simulink model "position_control"  (R2021a)
settings: Solver=ode23t  StartTime=0.0  StopTime=200  RelTol=1e-5
values from neighbouring files (symbols this model uses):
  g = 9.81    [quad_params.m]
  I = [     0.005831943165131                   0                   0 ... (first row only)    [quad_params.m]
  Kd_rates = [0.05,0.05,0.1]'    [quad_params.m]
  Kd_vel = [0.8,0.8,0.3]'    [quad_params.m]
  Ki_vel = [0.1,0.1,0.1]'    [quad_params.m]
  km = 1.2e-7    (= 1.2e-07)    [quad_params.m]
  Kp_att = [6,6,6]'    [quad_params.m]
  Kp_pos = [7,7,3]'    [quad_params.m]
  Kp_rates = [10,10,10]'    [quad_params.m]
  Kp_vel = [3,3,5]'    [quad_params.m]
  kt = 0.9e-5    (= 9e-06)    [quad_params.m]
  L = 0.2    [quad_params.m]
  m = 0.9272    [quad_params.m]
  q_init = [1;0;0;0]    [quad_params.m]
  rate_p_max = 3.5    [quad_params.m]
  thrust_max = thrust_max_per_motor*4    (= 32)    [quad_params.m]
  thrust_max_per_motor = 8    [quad_params.m]
  tilt_max = pi/6    (= 0.523598775598)    [quad_params.m]
  TQ_max_per_motor = km*(w_max.^2)    [quad_params.m]
  Vb_init = [0;0;0]    [quad_params.m]
  vel_xy_max = 15    [quad_params.m]
  vel_z_max = 10    [quad_params.m]
  wb_init = [0;0;0]    [quad_params.m]
  Xe_init = [0;0;0]    [quad_params.m]
undefined symbols (not defined in the file or in its folder): pm_0, sigbuilder_block, Vm_0, X, xme_0, Y, Z
libraries: simulink_extras x16, nesl_utility x5, aerolibutil x4, sm_lib x4, simulink x3, pid_lib x3, sharedtransform x3, sharedutil x1, vrlib x1, aerolibanim x1
(part 1 of 3)
settings Model: Creator=Petronas-Tareq  LastModifiedBy=Petronas-Tareq
settings SolverCC: AutoInsertRateTranBlk=on  InsertRTBMode=Always

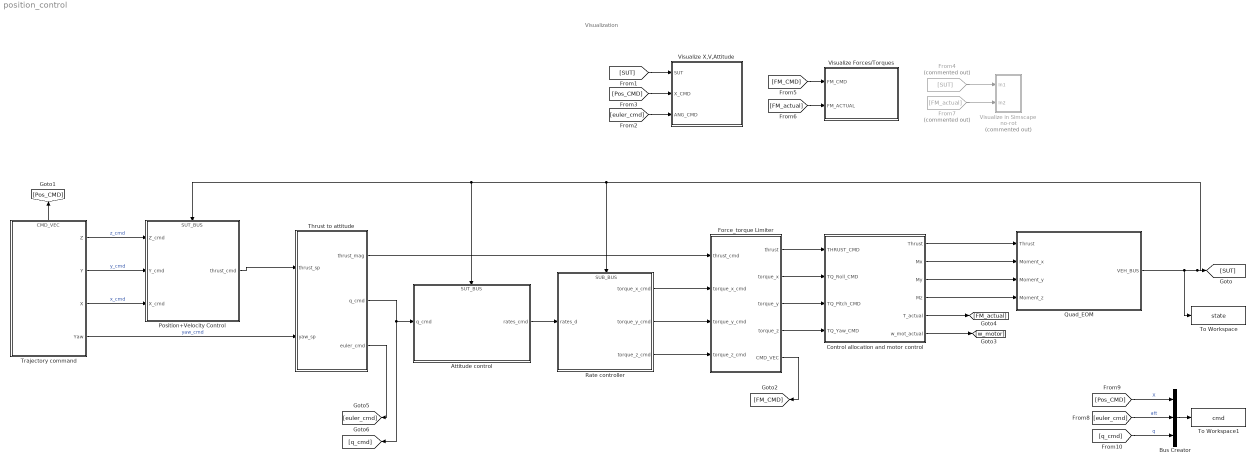
== system position_control ==
  note: Visualization
  Attitude control : Subsystem
      settings: PortSchema="{\"entries\":[{\"content\":{\"sides\":[{\"content\":{\"connectorIds\":[\"In1\"]},\"type\":\"ConnectorPlacement.EquallySpacedRectSide\",\"uuid\":\"19a574f6-5314-4727-8968-5b1c9712010e\"},{\"content\":{\"connectorIds\":[\"Out1\"],\"side\":\"RIGHT\"},\"type\":\"ConnectorPlacement.EquallySpacedRectSide\",\"uuid\":\"5cd6813f-6e17-48c1-918b-7c366c6d9cfa\"},{\"content\":{\"connectorIds\":[\"In2\"],\"side\":\"TOP\"},\"type\":\"ConnectorPlacement.EquallySpacedRectSide\",\"uuid\":\"b2bca67c-c4f4-4722-89a0-a16251073bfd\"}]},\"type\":\"ConnectorPlacement.EquallySpacedConnector\",\"uuid\":\"dcbf54f5-c136-40d5-a3db-9d2776e5196c\"}],\"packageUris\":[\"http://schema.mathworks.com/mf0/Connector/R2020b\"],\"version\":\"1.0\"}"
      mask Display: image('$imagefile'); % Use "Edit Image" on toolstrip to change.
  Bus Creator : BusCreator  Inputs=3
  Control allocation and motor control : Subsystem  Variant=on  VariantControlMode=label  LabelModeActiveChoice=Choice1
      mask Display: image('$imagefile'); % Use "Edit Image" on toolstrip to change.
  Force_torque Limiter : Subsystem
  From4 : From  Commented=on  GotoTag=SUT
  From7 : From  Commented=on  GotoTag=FM_actual
  Position+Velocity Control : Subsystem
      settings: PortSchema="{\"entries\":[{\"content\":{\"sides\":[{\"content\":{\"connectorIds\":[\"In1\",\"In2\",\"In3\"]},\"type\":\"ConnectorPlacement.EquallySpacedRectSide\",\"uuid\":\"cfe37ea9-b8e2-443a-9d65-596f0fda79c9\"},{\"content\":{\"connectorIds\":[\"Out1\"],\"side\":\"RIGHT\"},\"type\":\"ConnectorPlacement.EquallySpacedRectSide\",\"uuid\":\"f39f64e1-4b16-444a-b7d2-95ecb1b2a6fa\"},{\"content\":{\"connectorIds\":[\"In4\"],\"side\":\"TOP\"},\"type\":\"ConnectorPlacement.EquallySpacedRectSide\",\"uuid\":\"52402c3a-f2ac-44cf-8c94-dbfc3f851d2b\"}]},\"type\":\"ConnectorPlacement.EquallySpacedConnector\",\"uuid\":\"0122f56a-2702-493b-af7d-a25e6b9e04ed\"}],\"packageUris\":[\"http://schema.mathworks.com/mf0/Connector/R2020b\"],\"version\":\"1.0\"}"
  Quad_EOM : Subsystem
      mask Display: image('$imagefile'); % Use "Edit Image" on toolstrip to change.
  Rate controller : Subsystem
      settings: PortSchema="{\"entries\":[{\"content\":{\"sides\":[{\"content\":{\"connectorIds\":[\"In1\"]},\"type\":\"ConnectorPlacement.EquallySpacedRectSide\",\"uuid\":\"0af60e35-7b10-4750-a6af-1a3d920b4771\"},{\"content\":{\"connectorIds\":[\"Out1\",\"Out2\",\"Out3\"],\"side\":\"RIGHT\"},\"type\":\"ConnectorPlacement.EquallySpacedRectSide\",\"uuid\":\"931b0f34-b3f1-4a41-949f-3d763eca3151\"},{\"content\":{\"connectorIds\":[\"In2\"],\"side\":\"TOP\"},\"type\":\"ConnectorPlacement.EquallySpacedRectSide\",\"uuid\":\"84fe42fa-07d1-4fd9-ad2f-8c6651eaa98c\"}]},\"type\":\"ConnectorPlacement.EquallySpacedConnector\",\"uuid\":\"f603d2ac-5c20-4a82-ba8b-1c7971d6778a\"}],\"packageUris\":[\"http://schema.mathworks.com/mf0/Connector/R2020b\"],\"version\":\"1.0\"}"
  Thrust to attitude : Subsystem
  To Workspace : ToWorkspace  VariableName=state  SaveFormat=Timeseries  SampleTime=-1
  To Workspace1 : ToWorkspace  VariableName=cmd  SaveFormat=Timeseries  SampleTime=-1
  Trajectory command : Subsystem  Variant=on  VariantControlMode=label  LabelModeActiveChoice=6
      settings: PortSchema="{\"entries\":[{\"content\":{\"sides\":[{\"content\":{\"connectorIds\":[]},\"type\":\"ConnectorPlacement.EquallySpacedRectSide\",\"uuid\":\"8b658e99-682c-4d99-9859-63a6cdcf875c\"},{\"content\":{\"connectorIds\":[\"Out1\",\"Out2\",\"Out3\",\"Out4\"],\"side\":\"RIGHT\"},\"type\":\"ConnectorPlacement.EquallySpacedRectSide\",\"uuid\":\"566e7e32-52b1-45cc-9bb3-5343461c1cc0\"},{\"content\":{\"connectorIds\":[\"Out5\"],\"side\":\"TOP\"},\"type\":\"ConnectorPlacement.EquallySpacedRectSide\",\"uuid\":\"4cb1ab19-6483-4408-b5f4-106b35038f17\"}]},\"type\":\"ConnectorPlacement.EquallySpacedConnector\",\"uuid\":\"dc7c82fc-432d-4c18-9829-e6c2b483f5a7\"}],\"packageUris\":[\"http://schema.mathworks.com/mf0/Connector/R2020b\"],\"version\":\"1.0\"}"
  Visualize Forces/Torques : Subsystem
  Visualize X,V,Attitude : Subsystem
  Visualize in Simscape no-rot : Subsystem  Commented=on
  wires:
  [FM_CMD] -> Visualize Forces/Torques/1(FM_CMD)
  Force_torque Limiter/5(CMD_VEC) -> [FM_CMD]
  [FM_actual] -> Visualize Forces/Torques/2(FM_ACTUAL)
  Trajectory command/2(Y) -> Position+Velocity Control/2(Y_cmd)  "y_cmd"
  [SUT] -> Visualize X,V,Attitude/1(SUT)
  [Pos_CMD] -> Visualize X,V,Attitude/2(X_CMD)
  Trajectory command/3(X) -> Position+Velocity Control/3(X_cmd)  "x_cmd"
  Control allocation and motor control/1(Thrust) -> Quad_EOM/1(Thrust)
  Control allocation and motor control/2(Mx) -> Quad_EOM/2(Moment_x)
  Control allocation and motor control/3(My) -> Quad_EOM/3(Moment_y)
  Control allocation and motor control/4(Mz) -> Quad_EOM/4(Moment_z)
  Control allocation and motor control/5(T_actual) -> [FM_actual]
  Control allocation and motor control/6(w_mot_actual) -> [w_motor]
  Trajectory command/1(Z) -> Position+Velocity Control/1(Z_cmd)  "z_cmd"
  [euler_cmd] -> Visualize X,V,Attitude/3(ANG_CMD)
  From4/1 -> Visualize in Simscape no-rot/1(In1)
  From7/1 -> Visualize in Simscape no-rot/2(In2)
  Force_torque Limiter/4(torque_z) -> Control allocation and motor control/4(TQ_Yaw_CMD)
  Force_torque Limiter/3(torque_y) -> Control allocation and motor control/3(TQ_Pitch_CMD)
  Force_torque Limiter/2(torque_x) -> Control allocation and motor control/2(TQ_Roll_CMD)
  Force_torque Limiter/1(thrust) -> Control allocation and motor control/1(THRUST_CMD)
  Thrust to attitude/1(thrust_mag) -> Force_torque Limiter/1(thrust_cmd)
  Rate controller/2(torque_y_cmd) -> Force_torque Limiter/3(torque_y_cmd)
  Rate controller/3(torque_z_cmd) -> Force_torque Limiter/4(torque_z_cmd)
  Rate controller/1(torque_x_cmd) -> Force_torque Limiter/2(torque_x_cmd)
  Attitude control/1(rates_cmd) -> Rate controller/1(rates_d)
  Trajectory command/5(CMD_VEC) -> [Pos_CMD]
  Bus Creator/1 -> To Workspace1/1
  [Pos_CMD] -> Bus Creator/1  "X"
  [euler_cmd] -> Bus Creator/2  "att"
  [q_cmd] -> Bus Creator/3  "q"
  Thrust to attitude/2(q_cmd) -> Attitude control/1(q_cmd), [q_cmd]
  Thrust to attitude/3(euler_cmd) -> [euler_cmd]
  Trajectory command/4(Yaw) -> Thrust to attitude/2(yaw_sp)  "yaw_cmd"
  Position+Velocity Control/1(thrust_cmd) -> Thrust to attitude/1(thrust_sp)
  Quad_EOM/1(VEH_BUS) -> To Workspace/1, Rate controller/2(SUB_BUS), Position+Velocity Control/4(SUT_BUS), Attitude control/2(SUT_BUS), [SUT]

== system position_control/Attitude control ==
  note: Attitude control (full attitude control, i.e. yaw+thrust)
  note: Attitude Error Calculation
  q_cmd : Inport
  SUT_BUS : Inport  Port=2
  Bus Selector3 : BusSelector  OutputSignals=q
  K_attitude : Gain  Gain=Kp_att
  MATLAB Function1 : MATLAB Function  TreatAsAtomicUnit=on
  Product : Product
  Quaternion Inverse : aerolibutil/Quaternion Inverse
  Quaternion multiply : aerolibutil/Quaternion Multiplication
  Selector1 : Selector  InputPortWidth=4  IndexOptions=Index vector (dialog)  Indices=1  OutputSizes=1
  Selector2 : Selector  InputPortWidth=4  IndexOptions=Index vector (dialog)  Indices=2:4  OutputSizes=1
  k : Gain  Gain=2
  rates_cmd : Outport  VectorParamsAs1DForOutWhenUnconnected=off
  wires:
  SUT_BUS/1 -> [SUT]
  q_cmd/1 -> Quaternion multiply/2  "q_d"
  [SUT] -> Bus Selector3/1
  Bus Selector3/1 -> Quaternion Inverse/1  "<q>"
  Product/1 -> k/1  "error"
  Selector1/1 -> MATLAB Function1/1(q0)  "q0"
  MATLAB Function1/1(y) -> Product/1
  Selector2/1 -> Product/2  "q_vec"
  Quaternion multiply/1 -> Selector2/1, Selector1/1  "qe"
  k/1 -> K_attitude/1
  Quaternion Inverse/1 -> Quaternion multiply/1
  K_attitude/1 -> rates_cmd/1  "rates_cmd"

== system position_control/Control allocation and motor control ==
  note: 1) Add Subsystem or Model blocks as valid variant choices.
      | 2) You cannot connect blocks at this level. At simulation, connectivity is automatically
      | determined, based on the active variant and port name matching.
  THRUST_CMD : Inport
  TQ_Roll_CMD : Inport  Port=2
  TQ_Pitch_CMD : Inport  Port=3
  TQ_Yaw_CMD : Inport  Port=4
  Ideal Actuators with allocation : Subsystem  VariantControl=Choice2
  Ideal Actuattion (direct transfer) : Subsystem  VariantControl=Choice1
  Thrust : Outport
  Mx : Outport  Port=2
  My : Outport  Port=3
  Mz : Outport  Port=4
  T_actual : Outport  Port=5
  w_mot_actual : Outport  Port=6

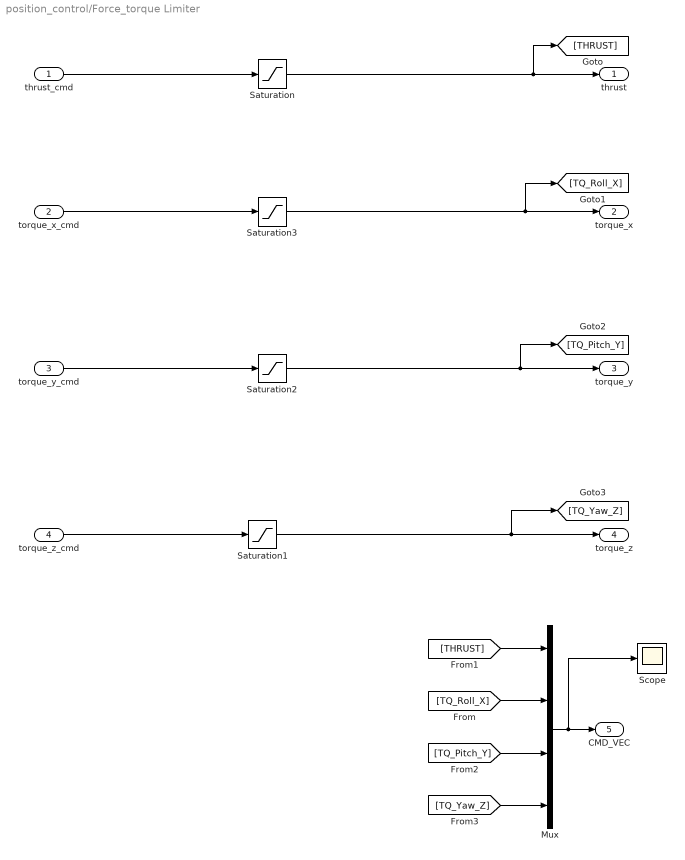
== system position_control/Force_torque Limiter ==
  thrust_cmd : Inport
  torque_x_cmd : Inport  Port=2
  torque_y_cmd : Inport  Port=3
  torque_z_cmd : Inport  Port=4
  Mux : Mux
  Saturation : Saturate  UpperLimit=thrust_max  LowerLimit=-thrust_max
      settings: AttributesFormatString=|
      | MAX =    %<UpperLimit>
      | MIN = %<LowerLimit>
  Saturation1 : Saturate  UpperLimit=2*TQ_max_per_motor  LowerLimit=-2*TQ_max_per_motor
      settings: AttributesFormatString=|
      | MAX =    %<UpperLimit>
      | MIN = %<LowerLimit>
  Saturation2 : Saturate  UpperLimit=thrust_max_per_motor*L  LowerLimit=-thrust_max_per_motor *L
      settings: AttributesFormatString=|
      | MAX =    %<UpperLimit>
      | MIN = %<LowerLimit>
  Saturation3 : Saturate  UpperLimit=thrust_max_per_motor*L  LowerLimit=-thrust_max_per_motor *L
      settings: AttributesFormatString=|
      | MAX =    %<UpperLimit>
      | MIN = %<LowerLimit>
  Scope : Scope
  thrust : Outport  VectorParamsAs1DForOutWhenUnconnected=off
  torque_x : Outport  Port=2  VectorParamsAs1DForOutWhenUnconnected=off
  torque_y : Outport  Port=3  VectorParamsAs1DForOutWhenUnconnected=off
  torque_z : Outport  Port=4  VectorParamsAs1DForOutWhenUnconnected=off
  CMD_VEC : Outport  Port=5  VectorParamsAs1DForOutWhenUnconnected=off
  wires:
  torque_z_cmd/1 -> Saturation1/1
  thrust_cmd/1 -> Saturation/1
  torque_y_cmd/1 -> Saturation2/1
  torque_x_cmd/1 -> Saturation3/1
  Saturation/1 -> [THRUST], thrust/1
  Saturation3/1 -> [TQ_Roll_X], torque_x/1
  Saturation2/1 -> [TQ_Pitch_Y], torque_y/1
  Saturation1/1 -> [TQ_Yaw_Z], torque_z/1
  Mux/1 -> Scope/1, CMD_VEC/1
  [THRUST] -> Mux/1
  [TQ_Roll_X] -> Mux/2
  [TQ_Pitch_Y] -> Mux/3
  [TQ_Yaw_Z] -> Mux/4

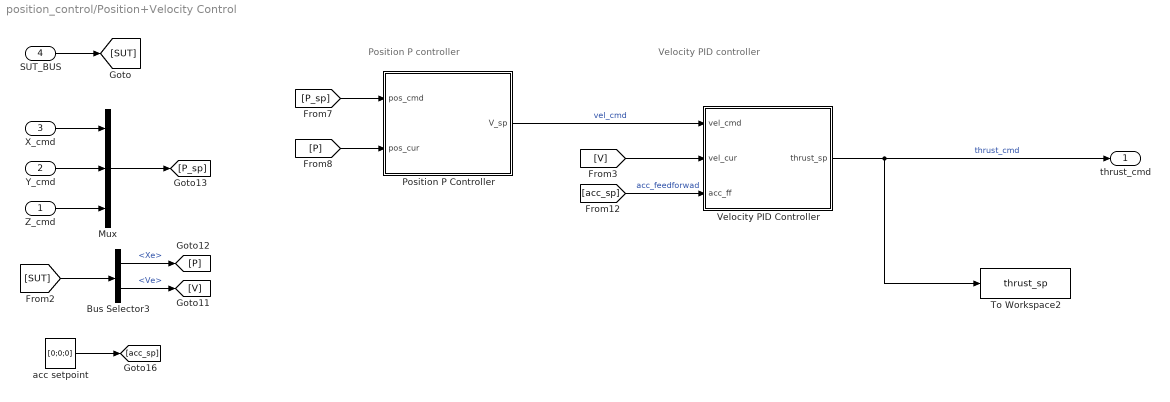
== system position_control/Position+Velocity Control ==
  note: Velocity PID controller
  note: Position P controller
  Z_cmd : Inport
  Y_cmd : Inport  Port=2
  X_cmd : Inport  Port=3
  SUT_BUS : Inport  Port=4
  Bus Selector3 : BusSelector  OutputSignals=Xe,Ve
  Mux : Mux  Inputs=3
  Position P Controller : Subsystem
  To Workspace2 : ToWorkspace  VariableName=thrust_sp  SaveFormat=Timeseries  SampleTime=-1
  Velocity PID Controller : Subsystem
  acc setpoint : Constant  Value=[0;0;0]
  thrust_cmd : Outport
  wires:
  SUT_BUS/1 -> [SUT]
  [SUT] -> Bus Selector3/1
  Bus Selector3/1 -> [P]  "<Xe>"
  Mux/1 -> [P_sp]
  acc setpoint/1 -> [acc_sp]
  [acc_sp] -> Velocity PID Controller/3(acc_ff)  "acc_feedforwad"
  Position P Controller/1(V_sp) -> Velocity PID Controller/1(vel_cmd)  "vel_cmd"
  [P_sp] -> Position P Controller/1(pos_cmd)
  [P] -> Position P Controller/2(pos_cur)
  [V] -> Velocity PID Controller/2(vel_cur)
  Velocity PID Controller/1(thrust_sp) -> To Workspace2/1, thrust_cmd/1  "thrust_cmd"
  Bus Selector3/2 -> [V]  "<Ve>"
  Z_cmd/1 -> Mux/3
  X_cmd/1 -> Mux/1
  Y_cmd/1 -> Mux/2

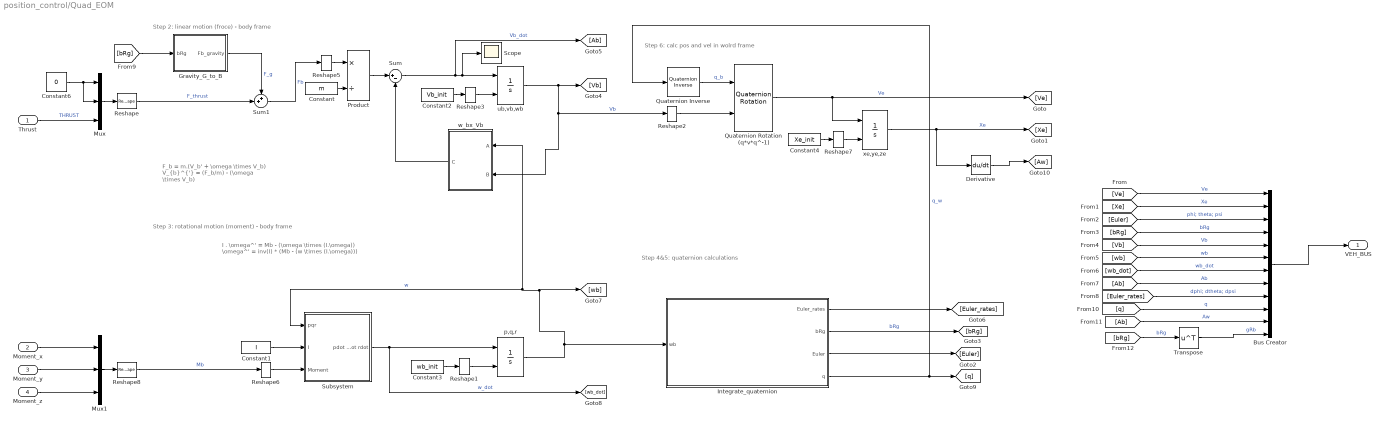
== system position_control/Quad_EOM ==
  note: Step 3: rotational motion (moment) - body frame
  note: F_b = m.(V_b' + \omega \times V_b)
      |
      | V_{b}^{'} = (F_b/m) - (\omega \times V_b)
  note: Step 2: linear motion (froce) - body frame
  note: Step 6: calc pos and vel in wolrd frame
  note: I . \omega^' = Mb - (\omega \times (I.\omega))
      |
      | \omega^' = inv(I) * (Mb - (w \times (I.\omega)))
  note: Step 4&5: quaternion calculations
  Thrust : Inport
  Moment_x : Inport  Port=2
  Moment_y : Inport  Port=3
  Moment_z : Inport  Port=4
  Bus Creator : BusCreator  Inputs=12
  Constant : Constant  Value=m  OutDataTypeStr=Inherit: Inherit via back propagation
  Constant1 : Constant  Value=I  OutDataTypeStr=Inherit: Inherit via back propagation
  Constant2 : Constant  Value=Vb_init  OutDataTypeStr=Inherit: Inherit via back propagation
  Constant3 : Constant  Value=wb_init  OutDataTypeStr=Inherit: Inherit via back propagation
  Constant4 : Constant  Value=Xe_init  OutDataTypeStr=Inherit: Inherit via back propagation
  Constant6 : Constant  Value=0
  Derivative : Derivative
  Gravity_G_to_B : Subsystem
  Integrate_quaternion : Subsystem
  Mux : Mux  Inputs=3
  Mux1 : Mux  Inputs=3
  Product : Product  Inputs=*/  SaturateOnIntegerOverflow=on  OutDataTypeStr=Inherit: Same as first input
  Quaternion Inverse : aerolibutil/Quaternion Inverse
  Quaternion Rotation (q*v*q^-1) : aerolibutil/Quaternion Rotation
  Reshape{,1..3,5..8} (8 alike) : Reshape  OutputDimensionality=Column vector (2-D)
  Scope : Scope
  Subsystem : Subsystem
  Sum : Sum  Inputs=|+-  SaturateOnIntegerOverflow=on
  Sum1 : Sum  Inputs=++|
  Transpose : Math  Operator=transpose  SaturateOnIntegerOverflow=on
  "p,q,r " : Integrator  InitialConditionSource=external  InitialCondition=pm_0
  ub,vb,wb : Integrator  InitialConditionSource=external  InitialCondition=Vm_0
  w_bx_Vb : Subsystem
      mask Display:
      | text(.5,.5,'Cross\nProduct\n\nC = AxB', ...
      | 	'HorizontalAlignment','Center',...
      | 	'VerticalAlignment','middle')
  xe,ye,ze : Integrator  InitialConditionSource=external  InitialCondition=xme_0
  VEH_BUS : Outport  VectorParamsAs1DForOutWhenUnconnected=off
  wires:
  [Euler] -> Bus Creator/3  "phi; theta; psi"
  [Xe] -> Bus Creator/2  "Xe"
  [Ve] -> Bus Creator/1  "Ve"
  [bRg] -> Bus Creator/4  "bRg"
  [Ab] -> Bus Creator/8  "Ab"
  [wb_dot] -> Bus Creator/7  "wb_dot"
  Bus Creator/1 -> VEH_BUS/1
  [Vb] -> Bus Creator/5  "Vb"
  [wb] -> Bus Creator/6  "wb"
  [Euler_rates] -> Bus Creator/9  "dphi; dtheta; dpsi"
  Reshape8/1 -> Reshape6/1  "Mb"
  Reshape6/1 -> Subsystem/3(Moment)
  Reshape1/1 -> "p,q,r "/2
  Constant2/1 -> Reshape3/1
  Subsystem/1(pdot qdot rdot) -> [wb_dot], "p,q,r "/1  "w_dot"
  Constant/1 -> Product/2
  Constant1/1 -> Subsystem/2(I)
  w_bx_Vb/1(C) -> Sum/2
  Integrate_quaternion/2(bRg) -> [bRg]  "bRg"
  Sum/1 -> [Ab], Scope/1, ub,vb,wb/1  "Vb_dot"
  Constant4/1 -> Reshape7/1
  Reshape3/1 -> ub,vb,wb/2
  Reshape7/1 -> xe,ye,ze/2
  Quaternion Rotation (q*v*q^-1)/1 -> xe,ye,ze/1, [Ve]  "Ve"
  Reshape5/1 -> Product/1
  xe,ye,ze/1 -> Derivative/1, [Xe]  "Xe"
  Sum1/1 -> Reshape5/1  "Fb"
  Constant3/1 -> Reshape1/1
  Product/1 -> Sum/1
  Constant6/1 -> Mux/2, Mux/1
  Gravity_G_to_B/1(Fb_gravity) -> Sum1/1  "F_g"
  Mux/1 -> Reshape/1
  Reshape/1 -> Sum1/2  "F_thrust"
  Thrust/1 -> Mux/3  "THRUST"
  [bRg] -> Gravity_G_to_B/1(bRg)
  Moment_y/1 -> Mux1/2
  Moment_z/1 -> Mux1/3
  Mux1/1 -> Reshape8/1
  Moment_x/1 -> Mux1/1
  "p,q,r "/1 -> [wb], Subsystem/1(pqr), w_bx_Vb/1(A), Integrate_quaternion/1(wb)  "w"
  ub,vb,wb/1 -> [Vb], w_bx_Vb/2(B), Reshape2/1  "Vb"
  Integrate_quaternion/1(Euler_rates) -> [Euler_rates]
  Integrate_quaternion/3(Euler) -> [Euler]
  [q] -> Bus Creator/10  "q"
  Integrate_quaternion/4(q) -> Quaternion Inverse/1, [q]  "q_w"
  Reshape2/1 -> Quaternion Rotation (q*v*q^-1)/2
  Quaternion Inverse/1 -> Quaternion Rotation (q*v*q^-1)/1  "q_b"
  Derivative/1 -> [Aw]
  [Ab] -> Bus Creator/11  "Aw"
  [bRg] -> Transpose/1  "bRg"
  Transpose/1 -> Bus Creator/12  "gRb"

== system position_control/Rate controller ==
  note: Rate controller
  rates_d : Inport
  SUB_BUS : Inport  Port=2
  Bus Selector1 : BusSelector  OutputSignals=wb,wb_dot
  Demux : Demux  Outputs=3
  Kd_rates : Gain  Gain=Kd_rates
  Kp_rates : Gain  Gain=Kp_rates
  Scope : Scope  NumInputPorts=2
  Sum : Sum  Inputs=|+-
  Sum1 : Sum  Inputs=|+-
  limit rate p : Saturate  UpperLimit=rate_p_max  LowerLimit=-rate_p_max
  limit rate q : Saturate  UpperLimit=rate_p_max  LowerLimit=-rate_p_max
  limit rate r : Saturate  UpperLimit=rate_p_max  LowerLimit=-rate_p_max
  torque_x_cmd : Outport
  torque_y_cmd : Outport  Port=2
  torque_z_cmd : Outport  Port=3
  wires:
  Bus Selector1/2 -> Kd_rates/1  "<wb_dot>"
  Bus Selector1/1 -> Sum1/2, Scope/2  "<wb>"
  Demux/1 -> limit rate p/1
  Demux/2 -> limit rate q/1
  Demux/3 -> limit rate r/1
  SUB_BUS/1 -> Bus Selector1/1  "measurements"
  rates_d/1 -> Sum1/1, Scope/1
  Kd_rates/1 -> Sum/2  "w_d"
  Kp_rates/1 -> Sum/1
  Sum/1 -> Demux/1  "torques"
  Sum1/1 -> Kp_rates/1
  limit rate p/1 -> torque_x_cmd/1
  limit rate q/1 -> torque_y_cmd/1
  limit rate r/1 -> torque_z_cmd/1

== system position_control/Thrust to attitude ==
  note: Thrust vector and Yaw to Attitude and total Thrust
  thrust_sp : Inport
  yaw_sp : Inport  Port=2
  Bus Creator : BusCreator  Inputs=3
  Demux4 : Demux  Outputs=3
  Direction Cosine Matrix to Quaternions : sharedtransform/Direction Cosine Matrix  to Quaternions  aMode=0  action=None  tolerance=eps(2)
      settings: SourceProductBaseCode=AE,PW,DR,MT,UV,VE
  MATLAB Function4 : MATLAB Function  TreatAsAtomicUnit=on
  Quaternions to Rotation Angles : sharedtransform/Quaternions to Rotation Angles  rotationOrder=ZYX  aMode=aMode
      settings: SourceProductBaseCode=AE,PW,DR,MT,UV,VE
  Scope1 : Scope
  Scope2 : Scope
  Subsystem : Subsystem  Commented=on
  To Workspace : ToWorkspace  VariableName=thrust_unit_dir  SaveFormat=Timeseries  SampleTime=-1
  To Workspace1 : ToWorkspace  VariableName=thrust_mag  SaveFormat=Timeseries  SampleTime=-1
  thrust_mag : Outport
  q_cmd : Outport  Port=2
  euler_cmd : Outport  Port=3
  wires:
  thrust_sp/1 -> Scope1/1, MATLAB Function4/1(thrust_sp)  "thrust_cmd"
  MATLAB Function4/1(R_sp) -> To Workspace/1, Direction Cosine Matrix to Quaternions/1
  MATLAB Function4/2(thrust_mag) -> thrust_mag/1, To Workspace1/1
  Direction Cosine Matrix to Quaternions/1 -> q_cmd/1, Quaternions to Rotation Angles/1
  yaw_sp/1 -> MATLAB Function4/2(yaw_sp)  "yaw_cmd"
  Demux4/1 -> Bus Creator/1  "yaw"
  Demux4/3 -> Bus Creator/3  "roll"
  Bus Creator/1 -> Scope2/1, euler_cmd/1
  Demux4/2 -> Bus Creator/2  "pitch"
  Quaternions to Rotation Angles/1 -> Demux4/1

== system position_control/Trajectory command ==
  Altitude : Subsystem  VariantControl=1
  Ground : Subsystem  VariantControl=0
  Position Trajectory : Subsystem  VariantControl=5
  Test to visualize thrust dir : Subsystem  VariantControl=6
  X Sine : Subsystem  VariantControl=4
  X ramp : Subsystem  VariantControl=9
  X square : Subsystem  VariantControl=7
  Y Sine : Subsystem  VariantControl=3
  Y ramp : Subsystem  VariantControl=8
  Yaw Sine : Subsystem  VariantControl=2
  Z : Outport
  Y : Outport  Port=2
  X : Outport  Port=3
  Yaw : Outport  Port=4
  CMD_VEC : Outport  Port=5

== system position_control/Visualize Forces//Torques ==
  FM_CMD : Inport
  FM_ACTUAL : Inport  Port=2
  FM CMD vs Actual : Scope  NumInputPorts=4
  FM_Mux : Subsystem
  wires:
  FM_CMD/1 -> [FM_CMD]
  [FM_CMD] -> FM_Mux/1(FM_CMD)
  [FM] -> FM_Mux/2(FM)
  FM_Mux/1(Y1) -> FM CMD vs Actual/1  "Thrust"
  FM_Mux/2(Y2) -> FM CMD vs Actual/2  "TQ_Roll_X"
  FM_Mux/3(w3) -> FM CMD vs Actual/3  "TQ_Pitch_Y"
  FM_Mux/4(Y4) -> FM CMD vs Actual/4  "TQ_Yaw_Z"
  FM_ACTUAL/1 -> [FM]

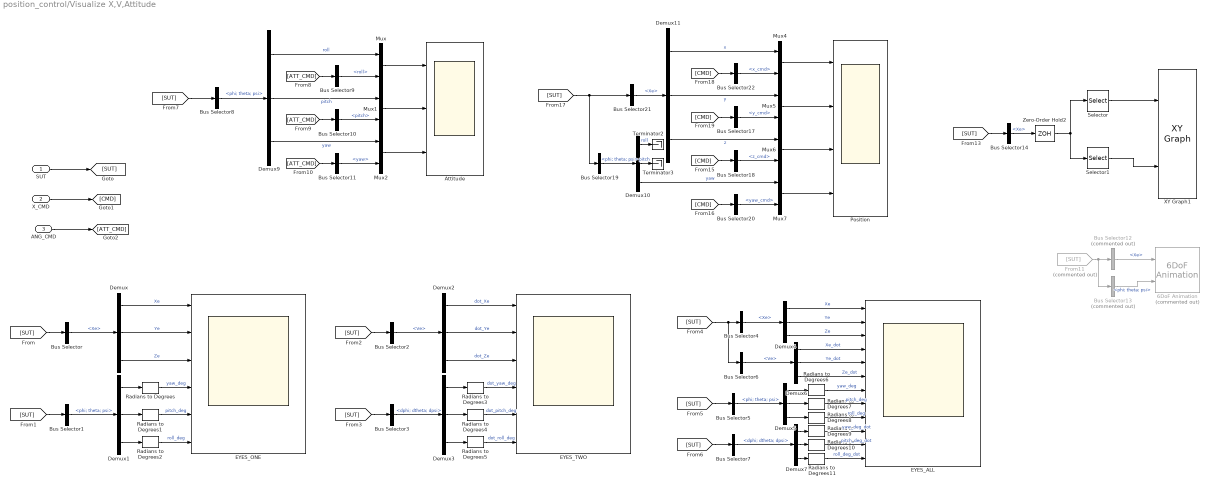
== system position_control/Visualize X,V,Attitude ==
  SUT : Inport
  X_CMD : Inport  Port=2
  ANG_CMD : Inport  Port=3
  6DoF Animation : aerolibanim/6DoF Animation  Commented=on  u1=[-20 20 -20 20 -20 20]  u2=0.05  u3=0.5  u4=[-5 -5 0 5]  u5=Fly alongside  u6=[0 0 0]  u7=10  u8=on
  "Attitude " : Scope  NumInputPorts=3
  Bus Selector{,4,14,21} (4 alike) : BusSelector  OutputSignals=Xe
  Bus Selector{1,5,8,19} (4 alike) : BusSelector  OutputSignals=phi; theta; psi
  Bus Selector10 : BusSelector  OutputSignals=pitch
  Bus Selector11 : BusSelector  OutputSignals=yaw
  Bus Selector12 : BusSelector  Commented=on  OutputSignals=Xe
  Bus Selector13 : BusSelector  Commented=on  OutputSignals=phi; theta; psi
  Bus Selector17 : BusSelector  OutputSignals=y_cmd
  Bus Selector18 : BusSelector  OutputSignals=z_cmd
  Bus Selector2 : BusSelector  OutputSignals=Ve
  Bus Selector20 : BusSelector  OutputSignals=yaw_cmd
  Bus Selector22 : BusSelector  OutputSignals=x_cmd
  Bus Selector3 : BusSelector  OutputSignals=dphi; dtheta; dpsi
  Bus Selector6 : BusSelector  OutputSignals=Ve
  Bus Selector7 : BusSelector  OutputSignals=dphi; dtheta; dpsi
  Bus Selector9 : BusSelector  OutputSignals=roll
  Demux{,1..7,9..11} (11 alike) : Demux  Outputs=3
  EYES_ALL : Scope  NumInputPorts=12
  EYES_ONE : Scope  NumInputPorts=6
  EYES_TWO : Scope  NumInputPorts=6
  From11 : From  Commented=on  GotoTag=SUT
  Mux{,1..2,4..7} (7 alike) : Mux  Inputs=2
  Position : Scope  NumInputPorts=4
  Radians to Degrees{,1..11} (12 alike) : simulink_extras/Transformations/Radians to Degrees
  Selector : Selector  InputPortWidth=3  IndexOptions=Index vector (dialog)  Indices=1  OutputSizes=1
  Selector1 : Selector  InputPortWidth=3  IndexOptions=Index vector (dialog)  Indices=2  OutputSizes=1
  Terminator2 : Terminator
  Terminator3 : Terminator
  XY Graph1 : simulink/Sinks/XY Graph  xmin=-1  xmax=30  ymin=-1  ymax=35  st=-1
  Zero-Order Hold2 : ZeroOrderHold  SampleTime=0.1
  wires:
  SUT/1 -> [SUT]
  [SUT] -> Bus Selector/1
  Demux/2 -> EYES_ONE/2  "Ye"
  Demux/3 -> EYES_ONE/3  "Ze"
  Demux/1 -> EYES_ONE/1  "Xe"
  Bus Selector/1 -> Demux/1  "<Xe>"
  Bus Selector1/1 -> Demux1/1  "<phi; theta; psi>"
  [SUT] -> Bus Selector1/1
  Demux1/1 -> Radians to Degrees/1
  Radians to Degrees/1 -> EYES_ONE/4  "yaw_deg"
  Radians to Degrees1/1 -> EYES_ONE/5  "pitch_deg"
  Radians to Degrees2/1 -> EYES_ONE/6  "roll_deg"
  Demux1/3 -> Radians to Degrees2/1
  Demux1/2 -> Radians to Degrees1/1
  [SUT] -> Bus Selector2/1
  Demux2/2 -> EYES_TWO/2  "dot_Ye"
  Demux2/3 -> EYES_TWO/3  "dot_Ze"
  Demux2/1 -> EYES_TWO/1  "dot_Xe"
  Bus Selector2/1 -> Demux2/1  "<Ve>"
  Bus Selector3/1 -> Demux3/1  "<dphi; dtheta; dpsi>"
  [SUT] -> Bus Selector3/1
  Demux3/1 -> Radians to Degrees3/1
  Radians to Degrees3/1 -> EYES_TWO/4  "dot_yaw_deg"
  Radians to Degrees4/1 -> EYES_TWO/5  "dot_pitch_deg"
  Radians to Degrees5/1 -> EYES_TWO/6  "dot_roll_deg"
  Demux3/3 -> Radians to Degrees5/1
  Demux3/2 -> Radians to Degrees4/1
  [SUT] -> Bus Selector6/1, Bus Selector4/1
  Demux4/2 -> EYES_ALL/2  "Ye"
  Demux4/3 -> EYES_ALL/3  "Ze"
  Demux4/1 -> EYES_ALL/1  "Xe"
  Bus Selector4/1 -> Demux4/1  "<Xe>"
  Bus Selector5/1 -> Demux5/1  "<phi; theta; psi>"
  [SUT] -> Bus Selector5/1
  Demux5/1 -> Radians to Degrees6/1
  Demux6/1 -> EYES_ALL/4  "Xe_dot"
  Demux6/2 -> EYES_ALL/5  "Ye_dot"
  Demux6/3 -> EYES_ALL/6  "Ze_dot"
  Demux5/3 -> Radians to Degrees8/1
  Demux5/2 -> Radians to Degrees7/1
  Bus Selector6/1 -> Demux6/1  "<Ve>"
  Radians to Degrees6/1 -> EYES_ALL/7  "yaw_deg"
  Radians to Degrees7/1 -> EYES_ALL/8  "pitch_deg"
  Radians to Degrees8/1 -> EYES_ALL/9  "roll_deg"
  Bus Selector7/1 -> Demux7/1  "<dphi; dtheta; dpsi>"
  [SUT] -> Bus Selector7/1
  Demux7/1 -> Radians to Degrees9/1
  Demux7/2 -> Radians to Degrees10/1
  Demux7/3 -> Radians to Degrees11/1
  Radians to Degrees9/1 -> EYES_ALL/10  "yaw_deg_dot"
  Radians to Degrees10/1 -> EYES_ALL/11  "pitch_deg_dot"
  Radians to Degrees11/1 -> EYES_ALL/12  "roll_deg_dot"
  X_CMD/1 -> [CMD]
  [SUT] -> Bus Selector8/1
  Demux9/2 -> Mux1/1  "pitch"
  Demux9/1 -> Mux/1  "roll"
  Bus Selector8/1 -> Demux9/1  "<phi; theta; psi>"
  Mux/1 -> "Attitude "/1
  Mux1/1 -> "Attitude "/2
  Mux2/1 -> "Attitude "/3
  Demux9/3 -> Mux2/1  "yaw"
  [ATT_CMD] -> Bus Selector9/1
  Bus Selector9/1 -> Mux/2  "<roll>"
  [ATT_CMD] -> Bus Selector10/1
  Bus Selector10/1 -> Mux1/2  "<pitch>"
  [ATT_CMD] -> Bus Selector11/1
  Bus Selector11/1 -> Mux2/2  "<yaw>"
  [SUT] -> Bus Selector14/1
  Bus Selector14/1 -> Zero-Order Hold2/1  "<Xe>"
  Zero-Order Hold2/1 -> Selector1/1, Selector/1
  Demux10/3 -> Mux7/1  "yaw"
  Mux7/1 -> Position/4
  Demux11/1 -> Mux4/1  "x"
  [CMD] -> Bus Selector20/1
  Bus Selector20/1 -> Mux7/2  "<yaw_cmd>"
  [CMD] -> Bus Selector17/1
  [SUT] -> Bus Selector21/1, Bus Selector19/1
  Demux10/2 -> Terminator3/1  "pitch"
  Mux6/1 -> Position/3
  Bus Selector19/1 -> Demux10/1  "<phi; theta; psi>"
  Demux10/1 -> Terminator2/1  "roll"
  Demux11/2 -> Mux5/1  "y"
  Bus Selector17/1 -> Mux5/2  "<y_cmd>"
  Mux4/1 -> Position/1
  Demux11/3 -> Mux6/1  "z"
  [CMD] -> Bus Selector22/1
  Mux5/1 -> Position/2
  Bus Selector22/1 -> Mux4/2  "<x_cmd>"
  Bus Selector18/1 -> Mux6/2  "<z_cmd>"
  [CMD] -> Bus Selector18/1
  Bus Selector21/1 -> Demux11/1  "<Xe>"
  ANG_CMD/1 -> [ATT_CMD]
  Selector/1 -> XY Graph1/1
  Selector1/1 -> XY Graph1/2
  From11/1 -> Bus Selector13/1, Bus Selector12/1
  Bus Selector12/1 -> 6DoF Animation/1  "<Xe>"
  Bus Selector13/1 -> 6DoF Animation/2  "<phi; theta; psi>"

== system position_control/Visualize in Simscape no-rot ==
  In1 : Inport
  In2 : Inport  Port=2
  6-DOF Joint1 : sm_lib/Joints/6-DOF Joint  JointMode=Normal  SenseConstraintForce=off  SenseConstraintForceX=off  SenseConstraintForceY=off  SenseConstraintForceZ=off  SenseConstraintTorque=off  SenseConstraintTorqueX=off  SenseConstraintTorqueY=off  SenseConstraintTorqueZ=off  SenseTotalForce=off  SenseTotalForceX=off  SenseTotalForceY=off  SenseTotalForceZ=off  SenseTotalTorque=off  SenseTotalTorqueX=off  SenseTotalTorqueY=off  SenseTotalTorqueZ=off  CompositeWrenchDir=FollowerOnBase  CompositeWrenchFrame=BaseFrame  PxEquilibriumPosition=0  PxEquilibriumPositionUnits=m  PxSpringStiffness=0  PxSpringStiffnessUnits=N/m  PxDampingCoefficient=0  PxDampingCoefficientUnits=N/(m/s)  PxTorqueActuationMode=ComputedTorque  PxMotionActuationMode=InputMotion  PxSensePosition=off  PxSenseVelocity=off  PxSenseAcceleration=off  PxSenseTorqueForce=off  PxSenseLowerLimitTorqueForce=off  PxSenseUpperLimitTorqueForce=off  PxLowerLimitSpecify=off  PxLowerLimitBound=-1  PxLowerLimitBoundUnits=m  PxLowerLimitStiffness=1e6  PxLowerLimitStiffnessUnits=N/m  PxLowerLimitDamping=1e3  PxLowerLimitDampingUnits=N/(m/s)  PxLowerLimitTransitionRegionWidth=1e-4  PxLowerLimitTransitionRegionWidthUnits=m  PxUpperLimitSpecify=off  PxUpperLimitBound=1  PxUpperLimitBoundUnits=m  PxUpperLimitStiffness=1e6  PxUpperLimitStiffnessUnits=N/m  PxUpperLimitDamping=1e3  PxUpperLimitDampingUnits=N/(m/s)  PxUpperLimitTransitionRegionWidth=1e-4  PxUpperLimitTransitionRegionWidthUnits=m  PxPositionTargetSpecify=on  PxPositionTargetPriority=High  PxPositionTargetValue=Xe_init(1)  PxPositionTargetValueUnits=m  PxVelocityTargetSpecify=off  PxVelocityTargetPriority=High  PxVelocityTargetValue=0  PxVelocityTargetValueUnits=m/s  PyEquilibriumPosition=0  PyEquilibriumPositionUnits=m  PySpringStiffness=0  PySpringStiffnessUnits=N/m  PyDampingCoefficient=0  PyDampingCoefficientUnits=N/(m/s)  PyTorqueActuationMode=ComputedTorque  PyMotionActuationMode=InputMotion  PySensePosition=off  PySenseVelocity=off  PySenseAcceleration=off  PySenseTorqueForce=off  PySenseLowerLimitTorqueForce=off  PySenseUpperLimitTorqueForce=off  PyLowerLimitSpecify=off  PyLowerLimitBound=-1  PyLowerLimitBoundUnits=m  PyLowerLimitStiffness=1e6  PyLowerLimitStiffnessUnits=N/m  PyLowerLimitDamping=1e3  PyLowerLimitDampingUnits=N/(m/s)  PyLowerLimitTransitionRegionWidth=1e-4  PyLowerLimitTransitionRegionWidthUnits=m  PyUpperLimitSpecify=off  PyUpperLimitBound=1  PyUpperLimitBoundUnits=m  PyUpperLimitStiffness=1e6  PyUpperLimitStiffnessUnits=N/m  PyUpperLimitDamping=1e3  PyUpperLimitDampingUnits=N/(m/s)  PyUpperLimitTransitionRegionWidth=1e-4  PyUpperLimitTransitionRegionWidthUnits=m  PyPositionTargetSpecify=on  PyPositionTargetPriority=High  PyPositionTargetValue=Xe_init(2)  PyPositionTargetValueUnits=m  PyVelocityTargetSpecify=off  PyVelocityTargetPriority=High  PyVelocityTargetValue=0  PyVelocityTargetValueUnits=m/s  PzEquilibriumPosition=0  PzEquilibriumPositionUnits=m  PzSpringStiffness=0  PzSpringStiffnessUnits=N/m  PzDampingCoefficient=0  PzDampingCoefficientUnits=N/(m/s)  PzTorqueActuationMode=ComputedTorque  PzMotionActuationMode=InputMotion  PzSensePosition=off  PzSenseVelocity=off  PzSenseAcceleration=off  PzSenseTorqueForce=off  PzSenseLowerLimitTorqueForce=off  PzSenseUpperLimitTorqueForce=off  PzLowerLimitSpecify=off  PzLowerLimitBound=-1  PzLowerLimitBoundUnits=m  PzLowerLimitStiffness=1e6  PzLowerLimitStiffnessUnits=N/m  PzLowerLimitDamping=1e3  PzLowerLimitDampingUnits=N/(m/s)  PzLowerLimitTransitionRegionWidth=1e-4  PzLowerLimitTransitionRegionWidthUnits=m  PzUpperLimitSpecify=off  PzUpperLimitBound=1  PzUpperLimitBoundUnits=m  PzUpperLimitStiffness=1e6  PzUpperLimitStiffnessUnits=N/m  PzUpperLimitDamping=1e3  PzUpperLimitDampingUnits=N/(m/s)  PzUpperLimitTransitionRegionWidth=1e-4  PzUpperLimitTransitionRegionWidthUnits=m  PzPositionTargetSpecify=on  PzPositionTargetPriority=High  PzPositionTargetValue=Xe_init(3)  PzPositionTargetValueUnits=m  PzVelocityTargetSpecify=off  PzVelocityTargetPriority=High  PzVelocityTargetValue=0  PzVelocityTargetValueUnits=m/s  SphDefPosRotationMethod=None  SphDefPosRotationAngleUnits=deg  SphDefPosRotationStandardAxis=+Z  SphDefPosRotationAngle=0.0  SphDefPosRotationArbitraryAxis=[0 0 1]  SphDefPosFollAlignAxisA=+X  SphDefPosBaseAlignAxisA=+Y  SphDefPosFollAlignAxisB=+Y  SphDefPosBaseAlignAxisB=+Z  SphDefPosRotationSequenceAxes=FollowerAxes  SphDefPosRotationSequence=XYX  SphDefPosRotationSequenceAngles=[0 0 0]  SphDefPosRotationSequenceAnglesUnits=deg  SphDefPosRotationMatrix=[1 0 0; 0 1 0; 0 0 1]  SphEqPosRotationMethod=None  SphEqPosRotationAngleUnits=deg  SphEqPosRotationStandardAxis=+Z  SphEqPosRotationAngle=0.0  SphEqPosRotationArbitraryAxis=[0 0 1]  SphEqPosFollAlignAxisA=+X  SphEqPosBaseAlignAxisA=+Y  SphEqPosFollAlignAxisB=+Y  SphEqPosBaseAlignAxisB=+Z  SphEqPosRotationSequenceAxes=FollowerAxes  SphEqPosRotationSequence=XYX  SphEqPosRotationSequenceAngles=[0 0 0]  SphEqPosRotationSequenceAnglesUnits=deg  SphEqPosRotationMatrix=[1 0 0; 0 1 0; 0 0 1]  SphSpringStiffness=0  SphSpringStiffnessUnits=N*m/deg  SphDampingCoefficient=0  SphDampingCoefficientUnits=N*m/(deg/s)  SphActuateTorqueX=off  SphActuateTorqueY=off  SphActuateTorqueZ=off  SphActuateTorque=on  SphTorqueActuationMode=InputTorque  SphMotionActuationMode=ComputedMotion  SphActuationFrame=BaseFrame  SphSensePosition=off  SphSenseVelocityX=off  SphSenseVelocityY=off  SphSenseVelocityZ=off  SphSenseVelocity=off  SphSenseAccelerationX=off  SphSenseAccelerationY=off  SphSenseAccelerationZ=off  SphSenseAcceleration=off  SphSenseTorqueX=off  SphSenseTorqueY=off  SphSenseTorqueZ=off  SphSenseTorqueForce=off  SphSenseLowerLimitTorqueMag=off  SphSenseUpperLimitTorqueMag=off  SphSensingFrame=BaseFrame  SphLowerLimitSpecify=off  SphLowerLimitBound=15  SphLowerLimitBoundUnits=deg  SphLowerLimitStiffness=1e4  SphLowerLimitStiffnessUnits=N*m/deg  SphLowerLimitDamping=10  SphLowerLimitDampingUnits=N*m/(deg/s)  SphLowerLimitTransitionRegionWidth=0.1  SphLowerLimitTransitionRegionWidthUnits=deg  SphUpperLimitSpecify=off  SphUpperLimitBound=45  SphUpperLimitBoundUnits=deg  SphUpperLimitStiffness=1e4  SphUpperLimitStiffnessUnits=N*m/deg  SphUpperLimitDamping=10  SphUpperLimitDampingUnits=N*m/(deg/s)  SphUpperLimitTransitionRegionWidth=0.1  SphUpperLimitTransitionRegionWidthUnits=deg  SphPositionTargetRotationMethod=RotationSequence  SphPositionTargetRotationAngleUnits=deg  SphPositionTargetRotationStandardAxis=+Z  SphPositionTargetRotationAngle=0.0  SphPositionTargetRotationArbitraryAxis=[0 0 1]  SphPositionTargetFollAlignAxisA=+X  SphPositionTargetBaseAlignAxisA=+Y  SphPositionTargetFollAlignAxisB=+Y  SphPositionTargetBaseAlignAxisB=+Z  SphPositionTargetRotationSequenceAxes=FollowerAxes  SphPositionTargetRotationSequence=ZYX  SphPositionTargetRotationSequenceAngles=eul_init  SphPositionTargetRotationSequenceAnglesUnits=rad  SphPositionTargetRotationMatrix=[1 0 0; 0 1 0; 0 0 1]  SphPositionTargetSpecify=on  SphPositionTargetPriority=High  SphVelocityTargetValue=0  SphVelocityTargetValueUnits=rad/s  SphVelocityTargetSpecify=off  SphVelocityTargetPriority=High  SphVelocityTargetInFollowerFrame=on
      settings: AttributesFormatString=|
      | %<PxPositionTargetValue> %<PyPositionTargetValue> %<PzPositionTargetValue>
      | %<PxVelocityTargetValue> %<PyVelocityTargetValue> %<PzVelocityTargetValue>
      | %<SphPositionTargetRotationSequenceAngles>
      | %<SphPositionTargetRotationSequence>
      | %<SphVelocityTargetValue>
  Bus Selector : BusSelector  OutputSignals=Xe
  Demux : Demux  Outputs=3
  Extruded Solid : sm_lib/Body Elements/Extruded Solid  GraphicAmbientColor=[0.15 0.15 0.15 1.0]  BasedOnType=Density  CenterOfMass=[0 0 0]  CenterOfMassUnits=m  GraphicDiffuseColor=[1.0 1.0 0.6]  ExportConvexHullGeometry=off  ExtrusionCrossSection=[1 1; -1 1; -1 -1; 1 -1]  ExtrusionCrossSectionUnits=m  Density=1000  DensityUnits=kg/m^3  DoExposeReferenceFrame=on  GraphicEmissiveColor=[0.0 0.0 0.0 1.0]  ExportEntireGeometry=off  ExtrusionLength=0.2  ExtrusionLengthUnits=m  ExtrusionType=Regular  SerializedFrames=<Frames/>  MarkerShape=Sphere  MarkerSize=10  GraphicType=FromGeometry  InertiaType=CalculateFromGeometry  Mass=1  MassUnits=kg  MomentsOfInertia=[1 1 1]  MomentsOfInertiaUnits=kg*m^2  PolygonNumSides=6  GraphicOpacity=1.0  PolygonOuterRadius=0.2  PolygonOuterRadiusUnits=m  ProductsOfInertia=[0 0 0]  ProductsOfInertiaUnits=kg*m^2  GraphicShininess=75  GraphicSpecularColor=[0.5 0.5 0.5 1.0]  GraphicVisPropType=SimpleVisualProperties
  Mechanism Configuration : sm_lib/Utilities/Mechanism Configuration  UniformGravity=Constant  GravityVector=[0, 0, -g]  GravityVectorUnits=m/s^2  GravityUnits=m/s^2  LinearizationDelta=0.001  JointModeTransitionNonlinearIterations=2
  Selector : Selector  InputPortWidth=4  IndexOptions=Index vector (dialog)  Indices=[2:4]  OutputSizes=1
  Simulink-PS Converter : nesl_utility/Simulink-PS Converter  PhysicalDomain=network_engine_domain  SubClassName=ps_input  LeftPortType=input  RightPortType=output  PseudoPeriodic=off  Frequencies=[]  NoiseDistribution=none  NoiseParameters=[]  Unit=m  AffineConversion=off  FilteringAndDerivatives=filter  SimscapeFilterOrder=2  InputFilterTimeConstant=0.001  UdotUserProvided=0
      settings: SourceProductBaseCode=PW,SS
  Simulink-PS Converter1 : nesl_utility/Simulink-PS Converter  PhysicalDomain=network_engine_domain  SubClassName=ps_input  LeftPortType=input  RightPortType=output  PseudoPeriodic=off  Frequencies=[]  NoiseDistribution=none  NoiseParameters=[]  Unit=m  AffineConversion=off  FilteringAndDerivatives=filter  SimscapeFilterOrder=2  InputFilterTimeConstant=0.001  UdotUserProvided=0
      settings: SourceProductBaseCode=PW,SS
  Simulink-PS Converter2 : nesl_utility/Simulink-PS Converter  PhysicalDomain=network_engine_domain  SubClassName=ps_input  LeftPortType=input  RightPortType=output  PseudoPeriodic=off  Frequencies=[]  NoiseDistribution=none  NoiseParameters=[]  Unit=m  AffineConversion=off  FilteringAndDerivatives=filter  SimscapeFilterOrder=2  InputFilterTimeConstant=0.001  UdotUserProvided=0
      settings: SourceProductBaseCode=PW,SS
  Simulink-PS Converter3 : nesl_utility/Simulink-PS Converter  PhysicalDomain=network_engine_domain  SubClassName=ps_input  LeftPortType=input  RightPortType=output  PseudoPeriodic=off  Frequencies=[]  NoiseDistribution=none  NoiseParameters=[]  Unit=N*m  AffineConversion=off  FilteringAndDerivatives=provide  SimscapeFilterOrder=1  InputFilterTimeConstant=0.001  UdotUserProvided=0
      settings: SourceProductBaseCode=PW,SS
  Solver Configuration : nesl_utility/Solver Configuration  PhysicalDomain=network_engine_domain  SubClassName=solver  LeftPortType=input  RightPortType=generic  Tones=[]  Harmonics=[]  SimulateNoise=off  Profile=off  UseLocalSampling=off  EnableSwitchedLinearOptims=on  FrequencyDomain=off  UseCCode=off  RelTol=0.001  AbsTol=1e-06  MinStep=1e-09  ToWorkspace=off  RevertToSquareIcSolve=off  NumHomotopyIterations=100  PhasorMode=off  PhasorModeNumHarmonics=1  DoDC=off  ResidualTolerance=1e-09  UseLocalSolver=off  LocalSolverChoice=NE_BACKWARD_EULER_ADVANCER  LocalSolverSampleTime=0.001  DoFixedCost=off  MaxNonlinIter=3  MaxModeIter=2  ComputeImpulses=off  ImpulseIterations=2  LinearAlgebra=Sparse  EquationFormulation=NE_TIME_EF  DelaysMemoryBudget=1024  AutomaticFiltering=on  FilteringTimeConstant=0.001  PartitionStorageMethod=AS_NEEDED  PartitionMemoryBudget=1024  PartitionMethod=FAST
  World Frame1 : sm_lib/Frames and Transforms/World Frame
  wires:
  Demux/3 -> Simulink-PS Converter2/1
  In2/1 -> Selector/1
  Demux/1 -> Simulink-PS Converter/1
  Selector/1 -> Simulink-PS Converter3/1
  Demux/2 -> Simulink-PS Converter1/1
  Bus Selector/1 -> Demux/1  "<Xe>"
  In1/1 -> Bus Selector/1
  connections:
  Simulink-PS Converter1/RConn1 -- 6-DOF Joint1/LConn3
  Solver Configuration/RConn1 -- 6-DOF Joint1/LConn1 -- Mechanism Configuration/RConn1 -- World Frame1/RConn1
  Simulink-PS Converter3/RConn1 -- 6-DOF Joint1/LConn5
  Simulink-PS Converter/RConn1 -- 6-DOF Joint1/LConn2
  Simulink-PS Converter2/RConn1 -- 6-DOF Joint1/LConn4
  Extruded Solid/RConn1 -- 6-DOF Joint1/RConn1

== system position_control/Control allocation and motor control/Ideal Actuators with allocation ==
  THRUST_CMD : Inport
  TQ_Roll_CMD : Inport  Port=2
  TQ_Pitch_CMD : Inport  Port=3
  TQ_Yaw_CMD : Inport  Port=4
  Control allocation : Subsystem
  Perfect actuators : Subsystem  VariantControl=Choice2
  Thrust : Outport
  Mx : Outport  Port=2
  My : Outport  Port=3
  Mz : Outport  Port=4
  T_actual : Outport  Port=5
  w_mot_actual : Outport  Port=6
  wires:
  Control allocation/1(w_command) -> Perfect actuators/1(w_cmd)
  THRUST_CMD/1 -> Control allocation/1(THRUST_CMD)
  TQ_Pitch_CMD/1 -> Control allocation/3(TQ_Pitch_CMD)
  TQ_Roll_CMD/1 -> Control allocation/2(TQ_Roll_CMD)
  TQ_Yaw_CMD/1 -> Control allocation/4(TQ_Yaw_CMD)
  Perfect actuators/5(T_actual) -> T_actual/1
  Perfect actuators/6(w_mot_actual) -> w_mot_actual/1
  Perfect actuators/3(My) -> My/1
  Perfect actuators/2(Mx) -> Mx/1
  Perfect actuators/4(Mz) -> Mz/1
  Perfect actuators/1(Thrust) -> Thrust/1

== system position_control/Control allocation and motor control/Ideal Actuattion (direct transfer) ==
  THRUST_CMD : Inport
  TQ_Roll_CMD : Inport  Port=2
  TQ_Pitch_CMD : Inport  Port=3
  TQ_Yaw_CMD : Inport  Port=4
  Mux : Mux
  Zero : Constant  Value=[0;0;0;0]  OutDataTypeStr=Inherit: Inherit via back propagation
  Thrust : Outport
  Mx : Outport  Port=2
  My : Outport  Port=3
  Mz : Outport  Port=4
  T_actual : Outport  Port=5
  w_mot_actual : Outport  Port=6
  wires:
  Zero/1 -> w_mot_actual/1
  TQ_Pitch_CMD/1 -> Mux/3, My/1
  TQ_Roll_CMD/1 -> Mux/2, Mx/1
  TQ_Yaw_CMD/1 -> Mux/4, Mz/1
  THRUST_CMD/1 -> Mux/1, Thrust/1
  Mux/1 -> T_actual/1

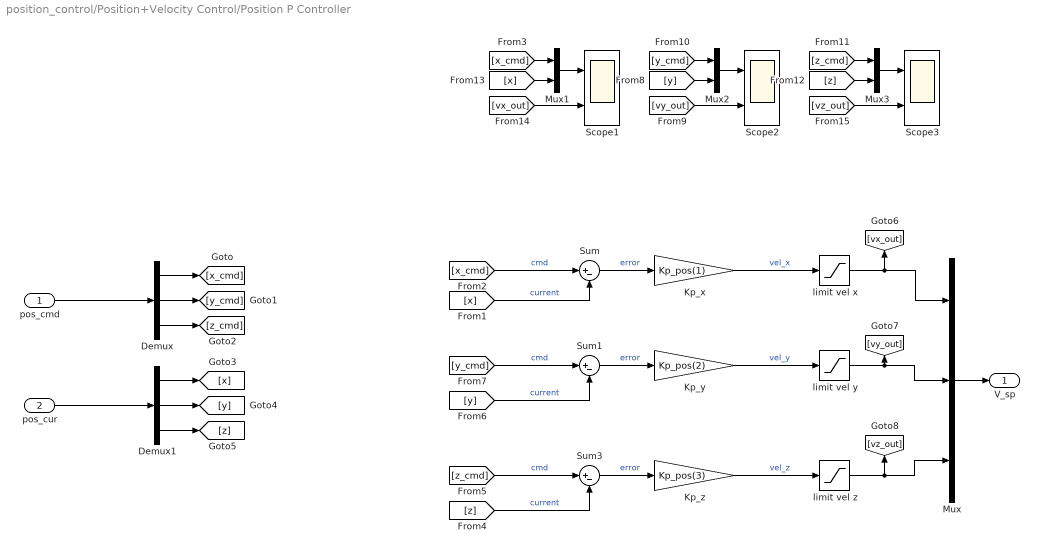
== system position_control/Position+Velocity Control/Position P Controller ==
  pos_cmd : Inport
  pos_cur : Inport  Port=2
  Demux : Demux  Outputs=3
  Demux1 : Demux  Outputs=3
  Kp_x : Gain  Gain=Kp_pos(1)
  Kp_y : Gain  Gain=Kp_pos(2)
  Kp_z : Gain  Gain=Kp_pos(3)
  Mux : Mux  Inputs=3
  Mux1 : Mux  Inputs=2
  Mux2 : Mux  Inputs=2
  Mux3 : Mux  Inputs=2
  Scope1 : Scope  NumInputPorts=2
  Scope2 : Scope  NumInputPorts=2
  Scope3 : Scope  NumInputPorts=2
  Sum : Sum  Inputs=|+-
  Sum1 : Sum  Inputs=|+-
  Sum3 : Sum  Inputs=|+-
  limit vel x : Saturate  UpperLimit=vel_xy_max  LowerLimit=-vel_xy_max
  limit vel y : Saturate  UpperLimit=vel_xy_max  LowerLimit=-vel_xy_max
  limit vel z : Saturate  UpperLimit=vel_z_max  LowerLimit=-vel_z_max
  V_sp : Outport
  wires:
  pos_cmd/1 -> Demux/1
  pos_cur/1 -> Demux1/1
  Demux/1 -> [x_cmd]
  Demux/2 -> [y_cmd]
  Demux/3 -> [z_cmd]
  Demux1/1 -> [x]
  Demux1/3 -> [z]
  Demux1/2 -> [y]
  [x_cmd] -> Sum/1  "cmd"
  Sum/1 -> Kp_x/1  "error"
  Mux/1 -> V_sp/1
  Kp_x/1 -> limit vel x/1  "vel_x"
  [x] -> Sum/2  "current"
  [z_cmd] -> Sum3/1  "cmd"
  [z] -> Sum3/2  "current"
  Sum3/1 -> Kp_z/1  "error"
  [y_cmd] -> Sum1/1  "cmd"
  [y] -> Sum1/2  "current"
  Sum1/1 -> Kp_y/1  "error"
  Kp_z/1 -> limit vel z/1  "vel_z"
  limit vel x/1 -> [vx_out], Mux/1
  Kp_y/1 -> limit vel y/1  "vel_y"
  limit vel y/1 -> [vy_out], Mux/2
  limit vel z/1 -> [vz_out], Mux/3
  [x_cmd] -> Mux1/1
  Mux1/1 -> Scope1/1
  [vx_out] -> Scope1/2
  [x] -> Mux1/2
  [y_cmd] -> Mux2/1
  Mux2/1 -> Scope2/1
  [vy_out] -> Scope2/2
  [y] -> Mux2/2
  [z_cmd] -> Mux3/1
  Mux3/1 -> Scope3/1
  [vz_out] -> Scope3/2
  [z] -> Mux3/2
